simulink model "NDI_AttitudeControl"  (R2021b)
settings: Solver=ode5  StartTime=0.0  StopTime=20  FixedStep=.005  RelTol=1e-3
values from neighbouring files (symbols this model uses):
  A_filt = [0 1; -wn^2 -2*zeta*wn]    [SetupModel.m]
  B_filt = [0;wn^2]    [SetupModel.m]
  C_filt = [eye(2);-wn^2 -2*zeta*wn]    [SetupModel.m]
  D_filt = [0;0;wn^2]    [SetupModel.m]
  dist = 300    [RunModel.m]    (also in SetupModel.m = 0)
  I = [Ixx 0 -Ixz; 0 Iyy 0; -Ixz 0 Izz]    [NDI_euler.m]    (also in SetupModel.m = [Ixx 0 -Ixz;0 Iyy 0; -Ixz 0 Izz])
  Im = I + diag(.15*diag(I))    [RunModel.m]    (also in SetupModel.m = I)
  K = [Kp Kd 0 0 0 0; 0 0 Kp Kd 0 0; 0 0 0 0 Kp Kd]    [NDI_euler.m]    (also in SetupModel.m = lqr(A,B,Q,R,[]))
  phi = 30*pi/180    (= 0.523598775598)    [SetupModel.m]
  phi0 = -25*pi/180    (= -0.436332312999)    [RunModel.m]    (also in SetupModel.m = 0)
  psi = 45*pi/180    (= 0.785398163397)    [SetupModel.m]
  psi0 = 15*pi/180    (= 0.261799387799)    [RunModel.m]    (also in SetupModel.m = 0)
  theta = -60*pi/180    (= -1.0471975512)    [SetupModel.m]
  theta0 = 20*pi/180    (= 0.349065850399)    [RunModel.m]    (also in SetupModel.m = 0)
  use_error_loop = 1    [RunModel.m]    (also in SetupModel.m = 0)
  x0 = [phi0 + phi_off;theta0 + theta;psi0 + psi_off;0;0;0]    [RunModel.m]    (also in SetupModel.m = [phi0;theta0;psi0;0;0;0])
libraries: matrix_library x2
settings Model: Creator=17165  LastModifiedBy=17165

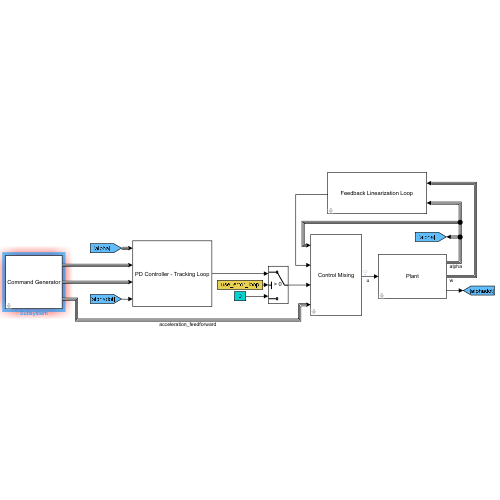
[thumbnail: Simulink's stored preview of the top-level diagram]
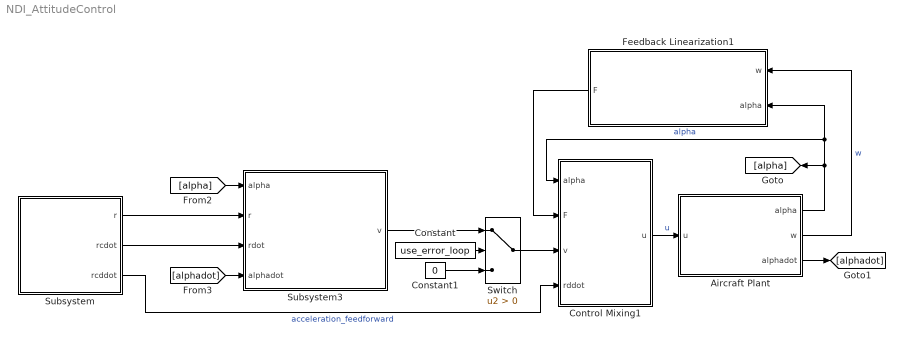
== system NDI_AttitudeControl ==
  Aircraft Plant : Subsystem  mask{I=I, x0=x0, dist=dist}
      mask prompts: I "Plant Moment of Inertia"; x0 "Initial Conditions"; dist "Disturbance Amplitude"
      mask Display: disp('Plant')
  Constant : Constant  Value=use_error_loop
  Constant1 : Constant  Value=0
  Control Mixing1 : Subsystem  mask{Im=Im}
      mask prompts: Im "Model Moment of Inertia"
      mask Display: disp('Control Mixing')
  Feedback Linearization1 : Subsystem  mask{Im=Im}
      mask prompts: Im "Model Moment of Inertia"
      mask Display: disp('Feedback Linearization Loop')
  Subsystem : Subsystem  mask{A=A_filt, B=B_filt, C=C_filt, D=D_filt, phic=phi, thetac=theta, psic=psi}
      mask prompts: A "Filter A"; B "Filter B"; C "Filter C"; D "Filter C"; phic "Roll command"; thetac "Pitch command"; psic "Roll command"
      mask Display: disp('Command Generator')
  Subsystem3 : Subsystem
      mask Display: disp('PD Controller - Tracking Loop')
  Switch : Switch  Criteria=u2 > Threshold
  wires:
  Subsystem/2(rcdot) -> Subsystem3/3(rdot)
  Subsystem3/1(v) -> Switch/1
  Subsystem/3(rcddot) -> Control Mixing1/4(rddot)  "acceleration_feedforward"
  Aircraft Plant/3(alphadot) -> [alphadot]
  Subsystem/1(r) -> Subsystem3/2(r)
  [alpha] -> Subsystem3/1(alpha)
  Constant1/1 -> Switch/3
  Aircraft Plant/1(alpha) -> Feedback Linearization1/2(alpha), Control Mixing1/1(alpha), [alpha]  "alpha"
  [alphadot] -> Subsystem3/4(alphadot)
  Control Mixing1/1(u) -> Aircraft Plant/1(u)  "u"
  Switch/1 -> Control Mixing1/3(v)
  Feedback Linearization1/1(F) -> Control Mixing1/2(F)
  Constant/1 -> Switch/2
  Aircraft Plant/2(w) -> Feedback Linearization1/1(w)  "w"

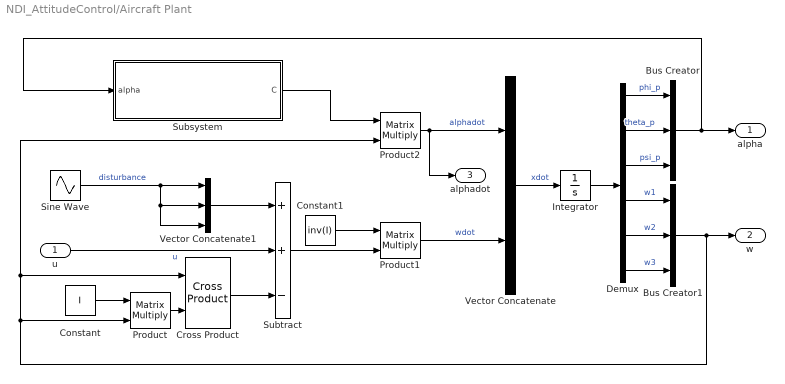
== system NDI_AttitudeControl/Aircraft Plant ==
  u : Inport
  Bus Creator : BusCreator  Inputs=3
  Bus Creator1 : BusCreator  Inputs=3
  Constant : Constant  Value=I
  Constant1 : Constant  Value=inv(I)
  Cross Product : matrix_library/Cross Product
      settings: SourceProductBaseCode=SL
  Demux : Demux  Outputs=6
  Integrator : Integrator  InitialCondition=x0
  Product : Product  Multiplication=Matrix(*)
  Product1 : Product  Multiplication=Matrix(*)
  Product2 : Product  Multiplication=Matrix(*)
  Sine Wave : Sin  Amplitude=dist  SampleTime=0
  Subsystem : Subsystem
      mask Display: disp('Inverse Kinematics Matrix: C')
  Subtract : Sum  Inputs=++-
  Vector Concatenate : Concatenate
  Vector Concatenate1 : Concatenate  NumInputs=3
  alpha : Outport
  w : Outport  Port=2
  alphadot : Outport  Port=3
  wires:
  Product/1 -> Cross Product/2
  Constant/1 -> Product/1
  Subtract/1 -> Product1/2
  Constant1/1 -> Product1/1
  Product1/1 -> Vector Concatenate/2  "wdot"
  Product2/1 -> alphadot/1, Vector Concatenate/1  "alphadot"
  Vector Concatenate/1 -> Integrator/1  "xdot"
  Integrator/1 -> Demux/1
  Demux/1 -> Bus Creator/1  "phi_p"
  Demux/3 -> Bus Creator/3  "psi_p"
  Demux/2 -> Bus Creator/2  "theta_p"
  Bus Creator/1 -> Subsystem/1(alpha), alpha/1
  Bus Creator1/1 -> Product2/2, Cross Product/1, Product/2, w/1
  Cross Product/1 -> Subtract/3
  u/1 -> Subtract/2  "u"
  Vector Concatenate1/1 -> Subtract/1
  Sine Wave/1 -> Vector Concatenate1/3, Vector Concatenate1/2, Vector Concatenate1/1  "disturbance"
  Demux/4 -> Bus Creator1/1  "w1"
  Demux/5 -> Bus Creator1/2  "w2"
  Demux/6 -> Bus Creator1/3  "w3"
  Subsystem/1(C) -> Product2/1

== system NDI_AttitudeControl/Control Mixing1 ==
  note: G = C*inv(I)
      | inv(G) = I*inv(C)
      |
      | u = inv(G)*(-F + rddot + v)
  alpha : Inport
  F : Inport  Port=2
  v : Inport  Port=3
  rddot : Inport  Port=4
  Add : Sum  Inputs=-++
  Gain1 : Gain  Gain=Im  Multiplication=Matrix(K*u)
  Matrix Divide : Product  Inputs=**  Multiplication=Matrix(*)
  Matrix Divide1 : Product  Inputs=/  Multiplication=Matrix(*)
  Subsystem : Subsystem
      mask Display: disp('Inverse Kinematics Matrix: C')
  u : Outport
  wires:
  F/1 -> Add/1
  rddot/1 -> Add/2
  v/1 -> Add/3
  Gain1/1 -> Matrix Divide/1
  Add/1 -> Matrix Divide/2
  Matrix Divide/1 -> u/1
  Matrix Divide1/1 -> Gain1/1
  Subsystem/1(C) -> Matrix Divide1/1
  alpha/1 -> Subsystem/1(alpha)

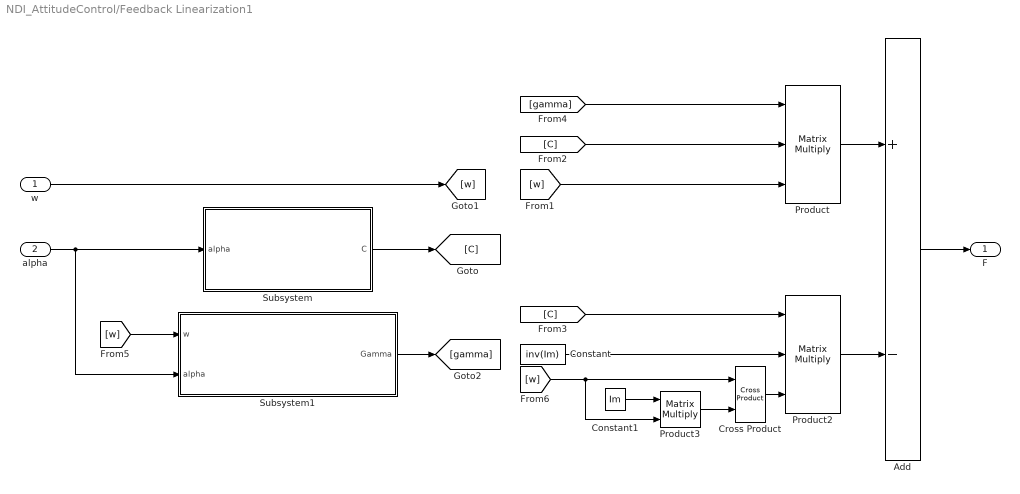
== system NDI_AttitudeControl/Feedback Linearization1 ==
  w : Inport
  alpha : Inport  Port=2
  Add : Sum  Inputs=+-
  Constant : Constant  Value=inv(Im)
  Constant1 : Constant  Value=Im
  Cross Product : matrix_library/Cross Product
      settings: SourceProductBaseCode=SL
  Product : Product  Inputs=3  Multiplication=Matrix(*)
  Product2 : Product  Inputs=3  Multiplication=Matrix(*)
  Product3 : Product  Multiplication=Matrix(*)
  Subsystem : Subsystem
      mask Display: disp('Inverse Kinematics Matrix: C')
  Subsystem1 : Subsystem
      mask Display: disp('Jacobian of Euler Angle Kinematics: gammma')
  F : Outport
  wires:
  alpha/1 -> Subsystem1/2(alpha), Subsystem/1(alpha)
  Subsystem/1(C) -> [C]
  [C] -> Product/2
  [w] -> Product/3
  [C] -> Product2/1
  Constant/1 -> Product2/2
  Constant1/1 -> Product3/1
  Product3/1 -> Cross Product/2
  Cross Product/1 -> Product2/3
  [w] -> Product3/2, Cross Product/1
  Product/1 -> Add/1
  Add/1 -> F/1
  Product2/1 -> Add/2
  Subsystem1/1(Gamma) -> [gamma]
  [gamma] -> Product/1
  w/1 -> [w]
  [w] -> Subsystem1/1(w)

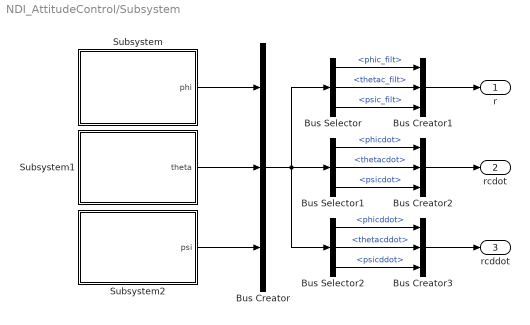
== system NDI_AttitudeControl/Subsystem ==
  Bus Creator{,1..3} (4 alike) : BusCreator  Inputs=3
  Bus Selector : BusSelector  OutputSignals=signal1.phic_filt,signal2.thetac_filt,signal3.psic_filt
  Bus Selector1 : BusSelector  OutputSignals=signal1.phicdot,signal2.thetacdot,signal3.psicdot
  Bus Selector2 : BusSelector  OutputSignals=signal1.phicddot,signal2.thetacddot,signal3.psicddot
  Subsystem : Subsystem  mask{A=A, B=B, C=C, D=D, amp=phic, IC=phi0}
      mask prompts: A "FIlter A Matrix"; B "Filter B Matrix"; C "Filter C Matrix"; D "Filter D Matrix"; amp "Euler Angle Command"; IC "Euler Angle IC"
      mask Display: disp('Filtered Command')
  Subsystem1 : Subsystem  mask{A=A, B=B, C=C, D=D, amp=thetac, IC=theta0}
      mask prompts: A "FIlter A Matrix"; B "Filter B Matrix"; C "Filter C Matrix"; D "Filter D Matrix"; amp "Euler Angle Command"; IC "Euler Angle IC"
      mask Display: disp('Filtered Command')
  Subsystem2 : Subsystem  mask{A=A, B=B, C=C, D=D, amp=psic, IC=psi0}
      mask prompts: A "FIlter A Matrix"; B "Filter B Matrix"; C "Filter C Matrix"; D "Filter D Matrix"; amp "Euler Angle Command"; IC "Euler Angle IC"
      mask Display: disp('Filtered Command')
  r : Outport
  rcdot : Outport  Port=2
  rcddot : Outport  Port=3
  wires:
  Subsystem/1(phi) -> Bus Creator/1
  Subsystem1/1(theta) -> Bus Creator/2
  Subsystem2/1(psi) -> Bus Creator/3
  Bus Creator1/1 -> r/1
  Bus Creator3/1 -> rcddot/1
  Bus Creator/1 -> Bus Selector2/1, Bus Selector1/1, Bus Selector/1
  Bus Selector/3 -> Bus Creator1/3  "<psic_filt>"
  Bus Selector/2 -> Bus Creator1/2  "<thetac_filt>"
  Bus Selector/1 -> Bus Creator1/1  "<phic_filt>"
  Bus Selector1/1 -> Bus Creator2/1  "<phicdot>"
  Bus Creator2/1 -> rcdot/1
  Bus Selector1/2 -> Bus Creator2/2  "<thetacdot>"
  Bus Selector1/3 -> Bus Creator2/3  "<psicdot>"
  Bus Selector2/1 -> Bus Creator3/1  "<phicddot>"
  Bus Selector2/3 -> Bus Creator3/3  "<psicddot>"
  Bus Selector2/2 -> Bus Creator3/2  "<thetacddot>"

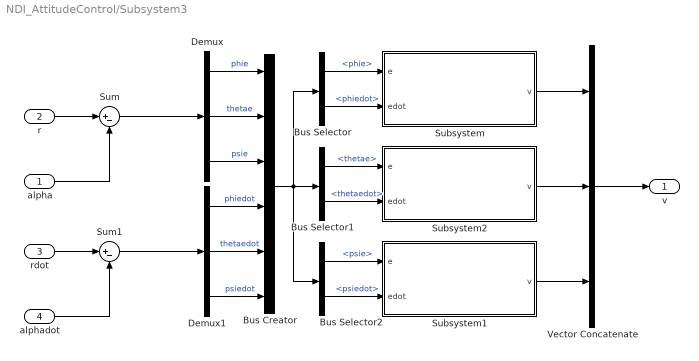
== system NDI_AttitudeControl/Subsystem3 ==
  alpha : Inport
  r : Inport  Port=2
  rdot : Inport  Port=3
  alphadot : Inport  Port=4
  Bus Creator : BusCreator  Inputs=6
  Bus Selector : BusSelector  OutputSignals=phie,phiedot
  Bus Selector1 : BusSelector  OutputSignals=thetae,thetaedot
  Bus Selector2 : BusSelector  OutputSignals=psie,psiedot
  Demux : Demux  Outputs=3
  Demux1 : Demux  Outputs=3
  Subsystem : Subsystem  mask{Kp=K(1), Kd=K(2)}
      mask Display: disp('PD-Compensator')
  Subsystem1 : Subsystem  mask{Kp=K(1), Kd=K(2)}
      mask Display: disp('PD-Compensator')
  Subsystem2 : Subsystem  mask{Kp=K(1), Kd=K(2)}
      mask Display: disp('PD-Compensator')
  Sum : Sum  Inputs=|+-
  Sum1 : Sum  Inputs=|+-
  Vector Concatenate : Concatenate  NumInputs=3
  v : Outport
  wires:
  Vector Concatenate/1 -> v/1
  Subsystem/1(v) -> Vector Concatenate/1
  Subsystem2/1(v) -> Vector Concatenate/2
  Subsystem1/1(v) -> Vector Concatenate/3
  Sum/1 -> Demux/1
  Sum1/1 -> Demux1/1
  Demux/1 -> Bus Creator/1  "phie"
  Demux/2 -> Bus Creator/2  "thetae"
  Demux/3 -> Bus Creator/3  "psie"
  Demux1/1 -> Bus Creator/4  "phiedot"
  Demux1/2 -> Bus Creator/5  "thetaedot"
  Demux1/3 -> Bus Creator/6  "psiedot"
  Bus Selector/1 -> Subsystem/1(e)  "<phie>"
  Bus Selector/2 -> Subsystem/2(edot)  "<phiedot>"
  Bus Selector2/2 -> Subsystem1/2(edot)  "<psiedot>"
  Bus Selector2/1 -> Subsystem1/1(e)  "<psie>"
  Bus Selector1/1 -> Subsystem2/1(e)  "<thetae>"
  Bus Selector1/2 -> Subsystem2/2(edot)  "<thetaedot>"
  Bus Creator/1 -> Bus Selector2/1, Bus Selector/1, Bus Selector1/1
  alpha/1 -> Sum/2
  r/1 -> Sum/1
  rdot/1 -> Sum1/1
  alphadot/1 -> Sum1/2

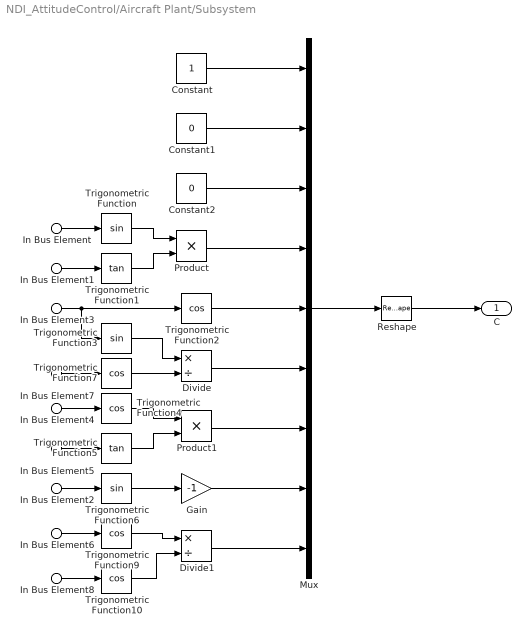
== system NDI_AttitudeControl/Aircraft Plant/Subsystem ==
  In Bus Element{1,5,7..8} (4 alike) : Inport  PortName=alpha  Element=theta_p
  In Bus Element{,2..4,6} (5 alike) : Inport  PortName=alpha  Element=phi_p
  Constant : Constant
  Constant1 : Constant  Value=0
  Constant2 : Constant  Value=0
  Divide : Product  Inputs=*/
  Divide1 : Product  Inputs=*/
  Gain : Gain  Gain=-1
  Mux : Mux  Inputs=9
  Product : Product
  Product1 : Product
  Reshape : Reshape  OutputDimensionality=Customize  OutputDimensions=[3,3]
  Trigonometric Function : Trigonometry
  Trigonometric Function1 : Trigonometry  Operator=tan
  Trigonometric Function{2,4,7,9..10} (5 alike) : Trigonometry  Operator=cos
  Trigonometric Function3 : Trigonometry
  Trigonometric Function5 : Trigonometry  Operator=tan
  Trigonometric Function6 : Trigonometry
  C : Outport
  wires:
  Constant/1 -> Mux/1
  Constant1/1 -> Mux/2
  Constant2/1 -> Mux/3
  In Bus Element/1 -> Trigonometric Function/1
  In Bus Element1/1 -> Trigonometric Function1/1
  Product/1 -> Mux/4
  Trigonometric Function/1 -> Product/1
  Trigonometric Function1/1 -> Product/2
  Trigonometric Function2/1 -> Mux/5
  Trigonometric Function4/1 -> Product1/1
  Product1/1 -> Mux/7
  Trigonometric Function5/1 -> Product1/2
  In Bus Element5/1 -> Trigonometric Function5/1
  In Bus Element4/1 -> Trigonometric Function4/1
  In Bus Element2/1 -> Trigonometric Function6/1
  Trigonometric Function6/1 -> Gain/1
  Gain/1 -> Mux/8
  Trigonometric Function3/1 -> Divide/1
  Divide/1 -> Mux/6
  Trigonometric Function7/1 -> Divide/2
  In Bus Element7/1 -> Trigonometric Function7/1
  In Bus Element3/1 -> Trigonometric Function3/1, Trigonometric Function2/1
  Trigonometric Function10/1 -> Divide1/2
  In Bus Element6/1 -> Trigonometric Function9/1
  Divide1/1 -> Mux/9
  In Bus Element8/1 -> Trigonometric Function10/1
  Trigonometric Function9/1 -> Divide1/1
  Mux/1 -> Reshape/1
  Reshape/1 -> C/1

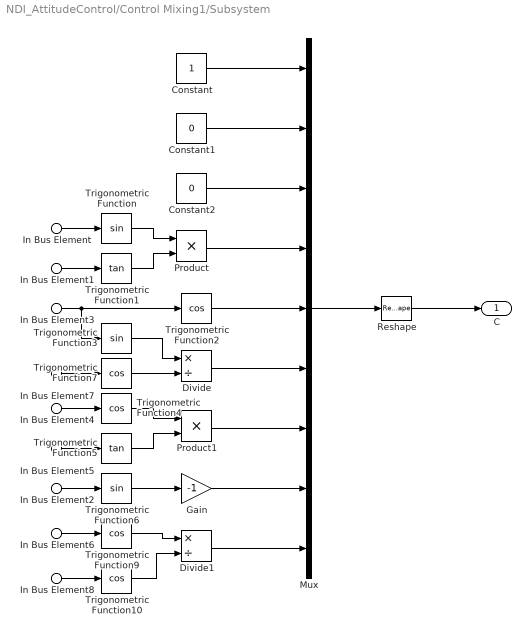
== system NDI_AttitudeControl/Control Mixing1/Subsystem ==
  In Bus Element{1,5,7..8} (4 alike) : Inport  PortName=alpha  Element=theta_p
  In Bus Element{,2..4,6} (5 alike) : Inport  PortName=alpha  Element=phi_p
  Constant : Constant
  Constant1 : Constant  Value=0
  Constant2 : Constant  Value=0
  Divide : Product  Inputs=*/
  Divide1 : Product  Inputs=*/
  Gain : Gain  Gain=-1
  Mux : Mux  Inputs=9
  Product : Product
  Product1 : Product
  Reshape : Reshape  OutputDimensionality=Customize  OutputDimensions=[3,3]
  Trigonometric Function : Trigonometry
  Trigonometric Function1 : Trigonometry  Operator=tan
  Trigonometric Function{2,4,7,9..10} (5 alike) : Trigonometry  Operator=cos
  Trigonometric Function3 : Trigonometry
  Trigonometric Function5 : Trigonometry  Operator=tan
  Trigonometric Function6 : Trigonometry
  C : Outport
  wires:
  Constant/1 -> Mux/1
  Constant1/1 -> Mux/2
  Constant2/1 -> Mux/3
  In Bus Element/1 -> Trigonometric Function/1
  In Bus Element1/1 -> Trigonometric Function1/1
  Product/1 -> Mux/4
  Trigonometric Function/1 -> Product/1
  Trigonometric Function1/1 -> Product/2
  Trigonometric Function2/1 -> Mux/5
  Trigonometric Function4/1 -> Product1/1
  Product1/1 -> Mux/7
  Trigonometric Function5/1 -> Product1/2
  In Bus Element5/1 -> Trigonometric Function5/1
  In Bus Element4/1 -> Trigonometric Function4/1
  In Bus Element2/1 -> Trigonometric Function6/1
  Trigonometric Function6/1 -> Gain/1
  Gain/1 -> Mux/8
  Trigonometric Function3/1 -> Divide/1
  Divide/1 -> Mux/6
  Trigonometric Function7/1 -> Divide/2
  In Bus Element7/1 -> Trigonometric Function7/1
  In Bus Element3/1 -> Trigonometric Function3/1, Trigonometric Function2/1
  Trigonometric Function10/1 -> Divide1/2
  In Bus Element6/1 -> Trigonometric Function9/1
  Divide1/1 -> Mux/9
  In Bus Element8/1 -> Trigonometric Function10/1
  Trigonometric Function9/1 -> Divide1/1
  Mux/1 -> Reshape/1
  Reshape/1 -> C/1

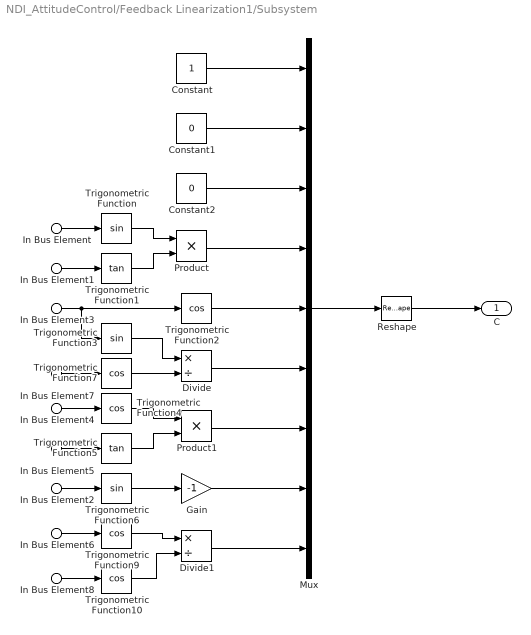
== system NDI_AttitudeControl/Feedback Linearization1/Subsystem ==
  In Bus Element{1,5,7..8} (4 alike) : Inport  PortName=alpha  Element=theta_p
  In Bus Element{,2..4,6} (5 alike) : Inport  PortName=alpha  Element=phi_p
  Constant : Constant
  Constant1 : Constant  Value=0
  Constant2 : Constant  Value=0
  Divide : Product  Inputs=*/
  Divide1 : Product  Inputs=*/
  Gain : Gain  Gain=-1
  Mux : Mux  Inputs=9
  Product : Product
  Product1 : Product
  Reshape : Reshape  OutputDimensionality=Customize  OutputDimensions=[3,3]
  Trigonometric Function : Trigonometry
  Trigonometric Function1 : Trigonometry  Operator=tan
  Trigonometric Function{2,4,7,9..10} (5 alike) : Trigonometry  Operator=cos
  Trigonometric Function3 : Trigonometry
  Trigonometric Function5 : Trigonometry  Operator=tan
  Trigonometric Function6 : Trigonometry
  C : Outport
  wires:
  Constant/1 -> Mux/1
  Constant1/1 -> Mux/2
  Constant2/1 -> Mux/3
  In Bus Element/1 -> Trigonometric Function/1
  In Bus Element1/1 -> Trigonometric Function1/1
  Product/1 -> Mux/4
  Trigonometric Function/1 -> Product/1
  Trigonometric Function1/1 -> Product/2
  Trigonometric Function2/1 -> Mux/5
  Trigonometric Function4/1 -> Product1/1
  Product1/1 -> Mux/7
  Trigonometric Function5/1 -> Product1/2
  In Bus Element5/1 -> Trigonometric Function5/1
  In Bus Element4/1 -> Trigonometric Function4/1
  In Bus Element2/1 -> Trigonometric Function6/1
  Trigonometric Function6/1 -> Gain/1
  Gain/1 -> Mux/8
  Trigonometric Function3/1 -> Divide/1
  Divide/1 -> Mux/6
  Trigonometric Function7/1 -> Divide/2
  In Bus Element7/1 -> Trigonometric Function7/1
  In Bus Element3/1 -> Trigonometric Function3/1, Trigonometric Function2/1
  Trigonometric Function10/1 -> Divide1/2
  In Bus Element6/1 -> Trigonometric Function9/1
  Divide1/1 -> Mux/9
  In Bus Element8/1 -> Trigonometric Function10/1
  Trigonometric Function9/1 -> Divide1/1
  Mux/1 -> Reshape/1
  Reshape/1 -> C/1

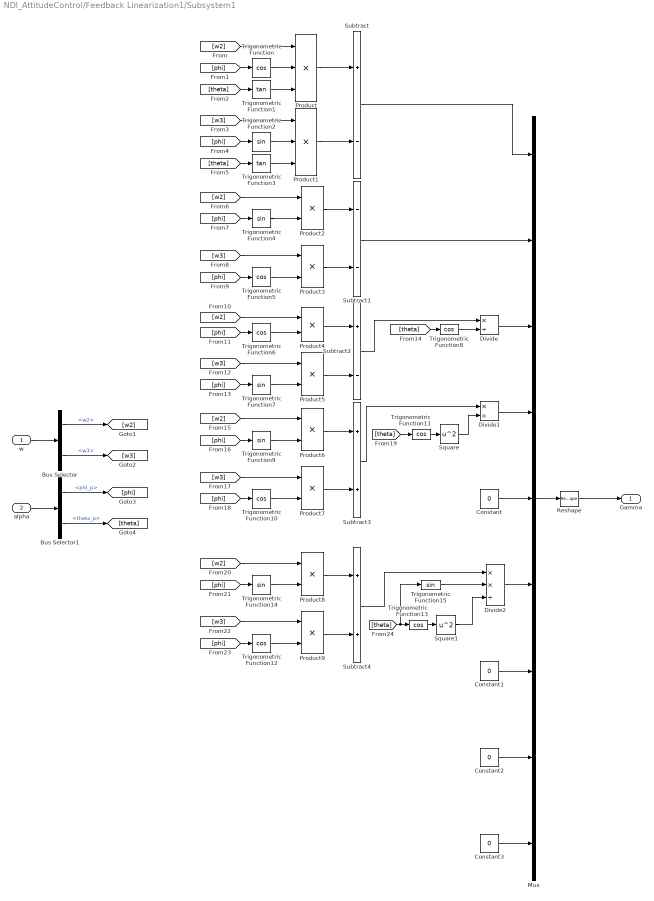
== system NDI_AttitudeControl/Feedback Linearization1/Subsystem1 ==
  w : Inport
  alpha : Inport  Port=2
  Bus Selector : BusSelector  OutputSignals=w2,w3
  Bus Selector1 : BusSelector  OutputSignals=phi_p,theta_p
  Constant{,1..3} (4 alike) : Constant  Value=0
  Divide : Product  Inputs=*/
  Divide1 : Product  Inputs=*/
  Divide2 : Product  Inputs=**/
  Mux : Mux  Inputs=9
  Product : Product  Inputs=3
  Product1 : Product  Inputs=3
  Product{2..9} (8 alike) : Product
  Reshape : Reshape  OutputDimensionality=Customize  OutputDimensions=[3,3]
  Square : Math  Operator=square  SaturateOnIntegerOverflow=on
  Square1 : Math  Operator=square  SaturateOnIntegerOverflow=on
  Subtract : Sum  Inputs=+-
  Subtract1 : Sum  Inputs=--
  Subtract2 : Sum  Inputs=+-
  Subtract3 : Sum
  Subtract4 : Sum
  Trigonometric Function{,5..6,8,10..13} (8 alike) : Trigonometry  Operator=cos
  Trigonometric Function1 : Trigonometry  Operator=tan
  Trigonometric Function{2,4,7,9,14..15} (6 alike) : Trigonometry
  Trigonometric Function3 : Trigonometry  Operator=tan
  Gamma : Outport
  wires:
  Subtract/1 -> Mux/1
  Mux/1 -> Reshape/1
  Reshape/1 -> Gamma/1
  w/1 -> Bus Selector/1
  Bus Selector/1 -> [w2]  "<w2>"
  Bus Selector/2 -> [w3]  "<w3>"
  alpha/1 -> Bus Selector1/1
  Bus Selector1/1 -> [phi]  "<phi_p>"
  Bus Selector1/2 -> [theta]  "<theta_p>"
  [w2] -> Product/1
  Trigonometric Function/1 -> Product/2
  [phi] -> Trigonometric Function/1
  Trigonometric Function1/1 -> Product/3
  [theta] -> Trigonometric Function1/1
  Product/1 -> Subtract/1
  Trigonometric Function3/1 -> Product1/3
  Product1/1 -> Subtract/2
  [theta] -> Trigonometric Function3/1
  Trigonometric Function2/1 -> Product1/2
  [w3] -> Product1/1
  [phi] -> Trigonometric Function2/1
  [phi] -> Trigonometric Function4/1
  Product2/1 -> Subtract1/1
  Trigonometric Function4/1 -> Product2/2
  Product3/1 -> Subtract1/2
  [w2] -> Product2/1
  Trigonometric Function5/1 -> Product3/2
  [phi] -> Trigonometric Function5/1
  [w3] -> Product3/1
  Subtract1/1 -> Mux/2
  [w3] -> Product5/1
  [phi] -> Trigonometric Function7/1
  Product4/1 -> Subtract2/1
  [w2] -> Product4/1
  [phi] -> Trigonometric Function6/1
  Trigonometric Function7/1 -> Product5/2
  Product5/1 -> Subtract2/2
  Trigonometric Function6/1 -> Product4/2
  Subtract2/1 -> Divide/1
  Divide/1 -> Mux/3
  Trigonometric Function8/1 -> Divide/2
  [theta] -> Trigonometric Function8/1
  Subtract3/1 -> Divide1/1
  [w3] -> Product7/1
  [phi] -> Trigonometric Function10/1
  Product6/1 -> Subtract3/1
  Trigonometric Function9/1 -> Product6/2
  [w2] -> Product6/1
  [phi] -> Trigonometric Function9/1
  Trigonometric Function10/1 -> Product7/2
  Product7/1 -> Subtract3/2
  [theta] -> Trigonometric Function11/1
  Divide1/1 -> Mux/4
  Trigonometric Function11/1 -> Square/1
  Square/1 -> Divide1/2
  Constant/1 -> Mux/5
  Constant3/1 -> Mux/9
  Constant2/1 -> Mux/8
  Constant1/1 -> Mux/7
  Product9/1 -> Subtract4/2
  Trigonometric Function12/1 -> Product9/2
  [phi] -> Trigonometric Function14/1
  Trigonometric Function14/1 -> Product8/2
  [w3] -> Product9/1
  [w2] -> Product8/1
  Trigonometric Function13/1 -> Square1/1
  [phi] -> Trigonometric Function12/1
  Product8/1 -> Subtract4/1
  Divide2/1 -> Mux/6
  Square1/1 -> Divide2/3
  Subtract4/1 -> Divide2/1
  Trigonometric Function15/1 -> Divide2/2
  [theta] -> Trigonometric Function15/1, Trigonometric Function13/1

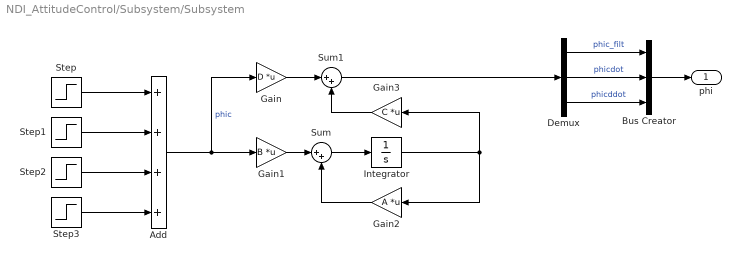
== system NDI_AttitudeControl/Subsystem/Subsystem ==
  Add : Sum  Inputs=++++
  Bus Creator : BusCreator  Inputs=3
  Demux : Demux  Outputs=3
  Gain : Gain  Gain=D  Multiplication=Matrix(K*u)
  Gain1 : Gain  Gain=B  Multiplication=Matrix(K*u)
  Gain2 : Gain  Gain=A  Multiplication=Matrix(K*u)
  Gain3 : Gain  Gain=C  Multiplication=Matrix(K*u)
  Integrator : Integrator  InitialCondition=[IC;0]
  Step : Step  Before=IC  After=amp  SampleTime=0
  Step1 : Step  Time=6  After=-amp  SampleTime=0
  Step2 : Step  Time=6  After=-amp  SampleTime=0
  Step3 : Step  Time=11  After=amp  SampleTime=0
  Sum : Sum  Inputs=|++
  Sum1 : Sum  Inputs=|++
  phi : Outport
  wires:
  Gain/1 -> Sum1/1
  Sum1/1 -> Demux/1
  Add/1 -> Gain/1, Gain1/1  "phic"
  Step2/1 -> Add/3
  Gain1/1 -> Sum/1
  Integrator/1 -> Gain2/1, Gain3/1
  Step1/1 -> Add/2
  Step/1 -> Add/1
  Gain3/1 -> Sum1/2
  Step3/1 -> Add/4
  Gain2/1 -> Sum/2
  Sum/1 -> Integrator/1
  Bus Creator/1 -> phi/1
  Demux/1 -> Bus Creator/1  "phic_filt"
  Demux/2 -> Bus Creator/2  "phicdot"
  Demux/3 -> Bus Creator/3  "phicddot"

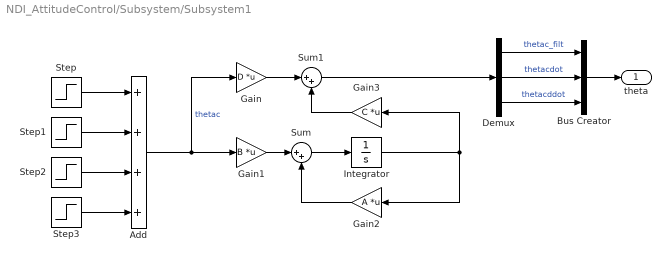
== system NDI_AttitudeControl/Subsystem/Subsystem1 ==
  Add : Sum  Inputs=++++
  Bus Creator : BusCreator  Inputs=3
  Demux : Demux  Outputs=3
  Gain : Gain  Gain=D  Multiplication=Matrix(K*u)
  Gain1 : Gain  Gain=B  Multiplication=Matrix(K*u)
  Gain2 : Gain  Gain=A  Multiplication=Matrix(K*u)
  Gain3 : Gain  Gain=C  Multiplication=Matrix(K*u)
  Integrator : Integrator  InitialCondition=[IC;0]
  Step : Step  Before=IC  After=amp  SampleTime=0
  Step1 : Step  Time=6  After=-amp  SampleTime=0
  Step2 : Step  Time=6  After=-amp  SampleTime=0
  Step3 : Step  Time=11  After=amp  SampleTime=0
  Sum : Sum  Inputs=|++
  Sum1 : Sum  Inputs=|++
  theta : Outport
  wires:
  Gain/1 -> Sum1/1
  Add/1 -> Gain/1, Gain1/1  "thetac"
  Step2/1 -> Add/3
  Gain1/1 -> Sum/1
  Integrator/1 -> Gain2/1, Gain3/1
  Step1/1 -> Add/2
  Step/1 -> Add/1
  Gain3/1 -> Sum1/2
  Step3/1 -> Add/4
  Gain2/1 -> Sum/2
  Sum/1 -> Integrator/1
  Demux/3 -> Bus Creator/3  "thetacddot"
  Demux/1 -> Bus Creator/1  "thetac_filt"
  Sum1/1 -> Demux/1
  Bus Creator/1 -> theta/1
  Demux/2 -> Bus Creator/2  "thetacdot"

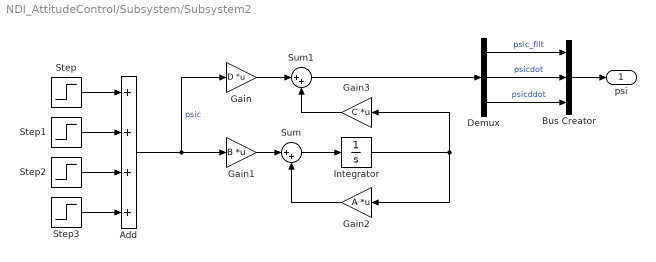
== system NDI_AttitudeControl/Subsystem/Subsystem2 ==
  Add : Sum  Inputs=++++
  Bus Creator : BusCreator  Inputs=3
  Demux : Demux  Outputs=3
  Gain : Gain  Gain=D  Multiplication=Matrix(K*u)
  Gain1 : Gain  Gain=B  Multiplication=Matrix(K*u)
  Gain2 : Gain  Gain=A  Multiplication=Matrix(K*u)
  Gain3 : Gain  Gain=C  Multiplication=Matrix(K*u)
  Integrator : Integrator  InitialCondition=[IC;0]
  Step : Step  Before=IC  After=amp  SampleTime=0
  Step1 : Step  Time=6  After=-amp  SampleTime=0
  Step2 : Step  Time=6  After=-amp  SampleTime=0
  Step3 : Step  Time=11  After=amp  SampleTime=0
  Sum : Sum  Inputs=|++
  Sum1 : Sum  Inputs=|++
  psi : Outport
  wires:
  Gain/1 -> Sum1/1
  Add/1 -> Gain/1, Gain1/1  "psic"
  Step2/1 -> Add/3
  Gain1/1 -> Sum/1
  Integrator/1 -> Gain2/1, Gain3/1
  Step1/1 -> Add/2
  Step/1 -> Add/1
  Gain3/1 -> Sum1/2
  Step3/1 -> Add/4
  Gain2/1 -> Sum/2
  Sum/1 -> Integrator/1
  Demux/3 -> Bus Creator/3  "psicddot"
  Demux/1 -> Bus Creator/1  "psic_filt"
  Sum1/1 -> Demux/1
  Bus Creator/1 -> psi/1
  Demux/2 -> Bus Creator/2  "psicdot"

== system NDI_AttitudeControl/Subsystem3/Subsystem ==
  e : Inport
  edot : Inport  Port=2
  Gain : Gain  Gain=Kp
  Gain1 : Gain  Gain=Kd
  Sum : Sum  Inputs=|++
  v : Outport
  wires:
  e/1 -> Gain/1
  Gain/1 -> Sum/1
  edot/1 -> Gain1/1
  Gain1/1 -> Sum/2
  Sum/1 -> v/1

== system NDI_AttitudeControl/Subsystem3/Subsystem1 ==
  e : Inport
  edot : Inport  Port=2
  Gain : Gain  Gain=Kp
  Gain1 : Gain  Gain=Kd
  Sum : Sum  Inputs=|++
  v : Outport
  wires:
  e/1 -> Gain/1
  Gain/1 -> Sum/1
  edot/1 -> Gain1/1
  Gain1/1 -> Sum/2
  Sum/1 -> v/1

== system NDI_AttitudeControl/Subsystem3/Subsystem2 ==
  e : Inport
  edot : Inport  Port=2
  Gain : Gain  Gain=Kp
  Gain1 : Gain  Gain=Kd
  Sum : Sum  Inputs=|++
  v : Outport
  wires:
  e/1 -> Gain/1
  Gain/1 -> Sum/1
  edot/1 -> Gain1/1
  Gain1/1 -> Sum/2
  Sum/1 -> v/1
